simulink model "frictionModelPaper"  (R2023b)
settings: Solver=FixedStepAuto  StartTime=0.0  StopTime=300  FixedStep=0.001  RelTol=1e-3
libraries: simulink x1
settings Model: Creator=snr  LastModifiedBy=snr

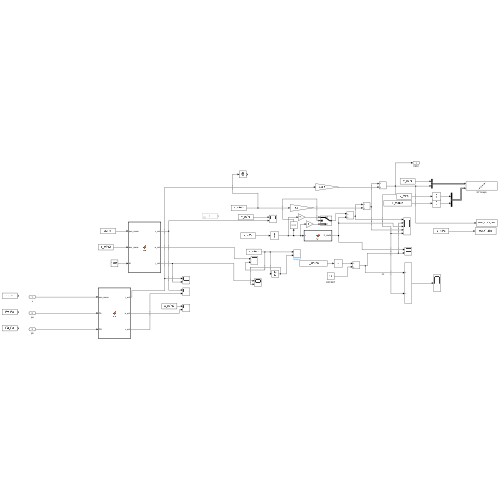
[thumbnail: Simulink's stored preview of the top-level diagram]
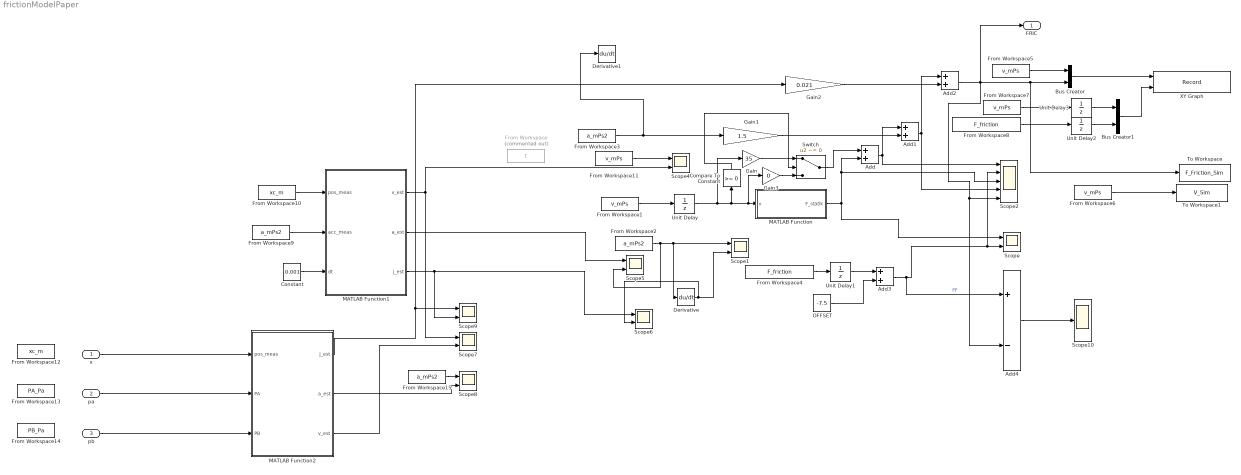
== system frictionModelPaper ==
  x : Inport
  pa : Inport  Port=2
  pb : Inport  Port=3
  Add{,1..3} (4 alike) : Sum
  Add4 : Sum  Inputs=+-
  Bus Creator : BusCreator  Inputs=2
  Bus Creator1 : BusCreator  Inputs=2
  Compare To Constant : simulink/Logic and Bit Operations/Compare To Constant  relop=>=  const=0  OutDataTypeStr=boolean
  Constant : Constant  Value=0.001
  Derivative : Derivative
  Derivative1 : Derivative
  From Workspace : FromWorkspace  Commented=on  VariableName=t
  From Workspace{1,5..7,11} (5 alike) : FromWorkspace  VariableName=v_mPs
  From Workspace10 : FromWorkspace  VariableName=xc_m
  From Workspace12 : FromWorkspace  VariableName=xc_m
  From Workspace13 : FromWorkspace  VariableName=PA_Pa
  From Workspace14 : FromWorkspace  VariableName=PB_Pa
  From Workspace{2..3,9,15} (4 alike) : FromWorkspace  VariableName=a_mPs2
  From Workspace4 : FromWorkspace  VariableName=F_friction
  From Workspace8 : FromWorkspace  VariableName=F_friction
  Gain : Gain  Gain=35
  Gain1 : Gain  Gain=1.5
  Gain2 : Gain  Gain=0.021
  Gain3 : Gain  Gain=0
  MATLAB Function : MATLAB Function  TreatAsAtomicUnit=on
  MATLAB Function1 : MATLAB Function  TreatAsAtomicUnit=on
  MATLAB Function2 : MATLAB Function  TreatAsAtomicUnit=on
  OFFSET : Constant  Value=-7.5
  Scope{,1,4..9} (8 alike) : Scope  NumInputPorts=2
  Scope10 : Scope
  Scope2 : Scope  NumInputPorts=5
  Switch : Switch  Criteria=u2 ~= 0  SaturateOnIntegerOverflow=off  InputSameDT=off
  To Workspace : ToWorkspace  VariableName=F_Friction_Sim  SaveFormat=Timeseries  SampleTime=-1
  To Workspace1 : ToWorkspace  VariableName=V_Sim  SaveFormat=Timeseries  SampleTime=-1
  Unit Delay{,1..3} (4 alike) : UnitDelay  SampleTime=-1  HasFrameUpgradeWarning=on
  XY Graph : Record  FileSettingsInternal="{\"entries\":[{\"content\":{\"excelSettings\":{\"content\":{},\"type\":\"Streamout.ExcelSettings\"}},\"type\":\"Streamout.FileSettingStorage\",\"uuid\":\"\"}],\"packageUris\":[\"http:\\/\\/schema.mathworks.com\\/mf0\\/streamout_blocks\\/R2020a\"],\"version\":\"1.0\"}"  Layout=[1 1]  SignalsInternal="{\"entries\":[{\"content\":{\"signals\":[{\"content\":{\"blockPath\":[],\"dimensions\":[1],\"domain\":\"\",\"hasChildren\":true,\"lineColor\":\"#fe330a\",\"port\":1,\"sid\":[\"\"],\"signalID\":7697,\"signalName\":\"Bus Creator\"},\"type\":\"RecordBlkView.Signal\",\"uuid\":\"\"},{\"content\":{\"blockPath\":[],\"dimensions\":[1],\"domain\":\"\",\"leafPath\":\"Bus Creator.signal1\",\"lineColor\":\"#fe330a\",\"parentID\":7697,\"plots\":[1],\"port\":1,\"sid\":[\"\"],\"signalID\":7703,\"signalName\":\"Bus Creator.signal1\"},\"type\":\"RecordBlkView.Signal\",\"uuid\":\"\"},{\"content\":{\"blockPath\":[],\"dimensions\":[1],\"domain\":\"\",\"leafPath\":\"Bus Creator.signal2\",\"lineColor\":\"#22b573\",\"parentID\":7697,\"plots\":[1],\"port\":1,\"sid\":[\"\"],\"signalID\":7707,\"signalName\":\"Bus Creator.signal2\"},\"type\":\"RecordBlkView.Signal\",\"uuid\":\"\"},{\"content\":{\"blockPath\":[],\"dimensions\":[1],\"domain\":\"\",\"hasChildren\":true,\"lineColor\":\"#d95319\",\"port\":2,\"sid\":[\"\"],\"signalID\":7709,\"signalName\":\"Bus Creator1\"},\"type\":\"RecordBlkView.Signal\",\"uuid\":\"\"},{\"content\":{\"blockPath\":[],\"dimensions\":[1],\"domain\":\"\",\"leafPath\":\"Bus Creator1.signal1\",\"lineColor\":\"#d95319\",\"parentID\":7709,\"plots\":[1],\"port\":2,\"sid\":[\"\"],\"signalID\":7715,\"signalName\":\"Bus Creator1.signal1\"},\"type\":\"RecordBlkView.Signal\",\"uuid\":\"\"},{\"content\":{\"blockPath\":[],\"dimensions\":[1],\"domain\":\"\",\"leafPath\":\"Bus Creator1.signal2\",\"lineColor\":\"#edb120\",\"parentID\":7709,\"plots\":[1],\"port\":2,\"sid\":[\"\"],\"signalID\":7719,\"signalName\":\"Bus Creator1.signal2\"},\"type\":\"RecordBlkView.Signal\",\"uuid\":\"\"}]},\"type\":\"RecordBlkView.InputSignals\",\"uuid\":\"\"}],\"packageUris\":[\"http:\\/\\/schema.mathworks.com\\/mf0\\/streamout_blocks\\/R2020a\"],\"version\":\"1.0\"}"  VisualizationBindings="{\"xyplotplugin\":{\"info\":[{\"series\":[{\"bindingParametersList\":[{\"parameter\":\"X-Axis\",\"signalID\":7715,\"signalName\":\"Bus Creator1.signal1\"},{\"parameter\":\"Y-Axis\",\"signalID\":7719,\"signalName\":\"Bus Creator1.signal2\"}],\"seriesID\":35013},{\"bindingParametersList\":[{\"parameter\":\"X-Axis\",\"signalID\":7703,\"signalName\":\"Bus Creator.signal1\"},{\"parameter\":\"Y-Axis\",\"signalID\":7707,\"signalName\":\"Bus Creator.signal2\"}],\"seriesID\":16995}],\"subplotID\":1}]}}"  CompatibilityTag=XY
  FRIC : Outport
  wires:
  From Workspace1/1 -> Unit Delay/1
  From Workspace2/1 -> Scope5/2, Scope1/1, Derivative/1
  MATLAB Function/1(F_statik) -> Add/2, Scope2/3, Scope/1
  From Workspace4/1 -> Unit Delay1/1
  Derivative/1 -> Scope6/2, Scope1/2
  Add/1 -> Add1/1, Scope2/1
  Gain1/1 -> Add1/2
  From Workspace3/1 -> Gain1/1, Derivative1/1
  Gain2/1 -> Add2/2
  Add1/1 -> Add2/1, Scope2/4
  Add2/1 -> FRIC/1, Add4/2, Scope2/5, Bus Creator/2, To Workspace/1
  MATLAB Function1/3(j_est) -> Scope9/2, Scope6/1
  From Workspace6/1 -> To Workspace1/1
  From Workspace5/1 -> Bus Creator/1
  Bus Creator/1 -> XY Graph/1
  From Workspace7/1 -> Unit Delay3/1
  From Workspace8/1 -> Unit Delay2/1
  Bus Creator1/1 -> XY Graph/2
  Unit Delay/1 -> Gain3/1, MATLAB Function/1(v), Compare To Constant/1, Gain/1
  Add3/1 -> Scope2/2, Scope/2, Add4/1  "FF"
  Unit Delay2/1 -> Bus Creator1/2
  Unit Delay3/1 -> Bus Creator1/1
  From Workspace9/1 -> MATLAB Function1/2(acc_meas)
  Constant/1 -> MATLAB Function1/3(dt)
  From Workspace10/1 -> MATLAB Function1/1(pos_meas)
  From Workspace11/1 -> Scope4/1
  MATLAB Function1/1(v_est) -> Scope7/1, Scope4/2
  MATLAB Function1/2(a_est) -> Scope5/1
  Unit Delay1/1 -> Add3/1
  OFFSET/1 -> Add3/2
  x/1 -> MATLAB Function2/1(pos_meas)
  pa/1 -> MATLAB Function2/2(PA)
  pb/1 -> MATLAB Function2/3(PB)
  MATLAB Function2/3(v_est) -> Scope7/2
  MATLAB Function2/2(a_est) -> Scope8/2
  From Workspace15/1 -> Scope8/1
  MATLAB Function2/1(j_est) -> Scope9/1, Gain2/1
  Add4/1 -> Scope10/1
  Compare To Constant/1 -> Switch/2
  Gain/1 -> Switch/1
  Gain3/1 -> Switch/3
  Switch/1 -> Add/1

== matlab function frictionModelPaper/MATLAB Function1 ==
  settings: updateMethod=DISCRETE
  data: pos_meas input; v_est output; acc_meas input; dt input; a_est output; j_est output
function [v_est, a_est, j_est] = fcn(pos_meas, acc_meas, dt)
    % KALMAN FİLTRESİ (Jerk Augmented)
    % Durumlar: x = [Pozisyon; Hız; İvme; Jerk]
    
    % Değişkenleri hafızada tutmak için 'persistent' tanımlıyoruz
    persistent x P A H Q R I initialized
    
    % --- BAŞLANGIÇ AYARLARI (Sadece ilk adımda çalışır) ---
    if isempty(initialized)
        % Başlangıç Durumu (İlk ölçüme göre)
        x = [pos_meas; 0; acc_meas; 0]; 
        
        % Başlangıç Belirsizliği
        P = eye(4); 
        
        % Matris Tanımları (Sabitler)
        % 1. Geçiş Matrisi (Fizik: x = x0 + v*dt + 0.5*a*dt^2 + ...)
        A = [1, dt, 0.5*dt^2, (1/6)*dt^3;
             0,  1,       dt,   0.5*dt^2;
             0,  0,        1,         dt;
             0,  0,        0,          1];
         
        % 2. Ölçüm Matrisi (Sadece Pos ve Acc ölçüyoruz)
        H = [1, 0, 0, 0;
             0, 0, 1, 0];
         
        % 3. Gürültü Kovaryansları (TUNING BURADAN)
        sigma_jerk = 2000; % Sistemin vahşiliği (Spike yakalama yeteneği)
        
        % Q (Süreç Gürültüsü)
        Q = diag([dt^6/36, dt^4/4, dt^2, 1]) * sigma_jerk^2;
        
        % R (Ölçüm Gürültüsü) - Sensör güveni
        R_pos = (1e-6)^2;
        R_acc = (0.5)^2;
        R = diag([R_pos, R_acc]);
        
        I = eye(4);
        initialized = 1;
    end
    
    % --- KALMAN DÖNGÜSÜ (Her adımda çalışır) ---
    
    % 1. PREDICT (Öngörü)
    x_pred = A * x;
    P_pred = A * P * A' + Q;
    
    % 2. UPDATE (Düzeltme)
    z = [pos_meas; acc_meas]; % Ölçüm vektörü
    
    y = z - H * x_pred;       % Innovation (Hata)
    S = H * P_pred * H' + R;  % Innovation Covaryans
    K = P_pred * H' / S;      % Kalman Kazancı
    
    x = x_pred + K * y;       % Durum Güncelleme
    P = (I - K * H) * P_pred; % Kovaryans Güncelleme
    
    % 3. ÇIKTI
    v_est = x(2);
    a_est = x(3);
    j_est = x(4);
end

== matlab function frictionModelPaper/MATLAB Function ==
  data: v input; F_statik output
function F_statik = fcn(v)
Fc = 18; 
Fs = 75; 
v_s = 0.016; 
C = 100; 

F_statik = Fc + (Fs - Fc)*exp(-(1*abs(v)./v_s)^2);
F_statik = F_statik * tanh(C*v);

== matlab function frictionModelPaper/MATLAB Function2 ==
  settings: updateMethod=DISCRETE
  data: j_est output; a_est output; pos_meas input; v_est output; PA input; PB input
function [j_est, a_est, v_est] = fcn(pos_meas, PA, PB)
    % PRESSURE-AIDED JERK ESTIMATOR
    % Girdiler: Pozisyon ve Basınçlar
    % Çıktı: Tertemiz Jerk (j_est)
    
    persistent x P A H Q R I initialized m AA AB
    
    % --- SABİTLER ---
    dt = 0.001;   % Örnekleme Zamanı (Simulink step size ile aynı olmalı)
    
    if isempty(initialized)
        % 1. SİSTEM TANIMLAMALARI
        m  = 3.4;       % Tahmini Hareketli Kütle (kg)
        AA = 2.0106e-04;  % A Odası Alanı (m2)
        AB = 2.0106e-04;  % B Odası Alanı (m2)
        
        % 2. DURUM VEKTÖRÜ: x = [Konum; Hız; İvme; Jerk]
        % (Sürtünme değil, doğrudan kinematiği izliyoruz)
        F_net_start = (PA*AA - PB*AB);
        a_start = F_net_start / m;
        
        x = [pos_meas; 0; a_start; 0];
        P = eye(4);
        I = eye(4);
        
        % 3. GEÇİŞ MATRİSİ (Constant Jerk Model)
        % x(k+1) = x(k) + v*dt + 0.5*a*dt^2 + 1/6*j*dt^3 ...
        A = [1, dt, 0.5*dt^2, (1/6)*dt^3;
             0,  1,       dt,   0.5*dt^2;
             0,  0,        1,         dt;
             0,  0,        0,          1];
         
        % 4. ÖLÇÜM MATRİSİ
        % z1 = Konum (x1)
        % z2 = İvme  (x3) -> Basınçtan türetilmiş "Sanal İvme"
        H = [1, 0, 0, 0;
             0, 0, 1, 0];
         
        % 5. TUNING (AYARLAR)
        % Q: Jerk ne kadar hızlı değişebilir? (Sistemin vahşiliği)
        % Yüksek değer = Zıplamaları anında yakalar (Gecikmesiz).
        sigma_jerk = 100; 
        Q = diag([dt^6/36, dt^4/4, dt^2, 1]) * sigma_jerk^2;
        
        % R: Ölçümlere ne kadar güveniyoruz?
        R_pos = (1e-6)^2; % Konum çok hassas
        R_acc = (2.0)^2;  % Basınçtan gelen ivme "gürültülüdür" (Sürtünme yok sayıldığı için)
                          % Burayı gevşek bırakıyoruz ki Kalman, konum verisiyle
                          % basınç verisini harmanlayıp doğruyu bulsun.
        R = diag([R_pos, R_acc]);
        
        initialized = 1;
    end
    
    % --- 1. SANAL İVME ÖLÇÜMÜ OLUŞTURMA ---
    % Basınç kuvvetini kütleye bölerek "Ham İvme" elde ediyoruz.
    % Not: Bu ivme sürtünmeyi içermez, bu yüzden "gürültülü/hatalı" kabul edilir.
    % Kalman bunu düzeltecek.
    F_hyd = PA * AA - PB * AB;
    a_meas_virtual = F_hyd / m; 
    
    % Ölçüm Vektörü
    z = [pos_meas; a_meas_virtual];
    
    % --- 2. KALMAN PREDICT ---
    x_pred = A * x;
    P_pred = A * P * A' + Q;
    
    % --- 3. KALMAN UPDATE ---
    y = z - H * x_pred;       % Hata (Innovation)
    S = H * P_pred * H' + R;  % Kovaryans
    K = P_pred * H' / S;      % Kazanç (Gain)
    
    x = x_pred + K * y;       % Güncelleme
    P = (I - K * H) * P_pred;
    
    % --- 4. ÇIKTILAR ---
    v_est = x(2);
    a_est = x(3);
    j_est = x(4); % İŞTE ARADIĞIN JERK!
end
